simulink model "DiagramaFase2"  (R2024b)
settings: Solver=VariableStepAuto  StartTime=0.0  StopTime=5  RelTol=1e-3
settings Model: Creator=david  LastModifiedBy=david

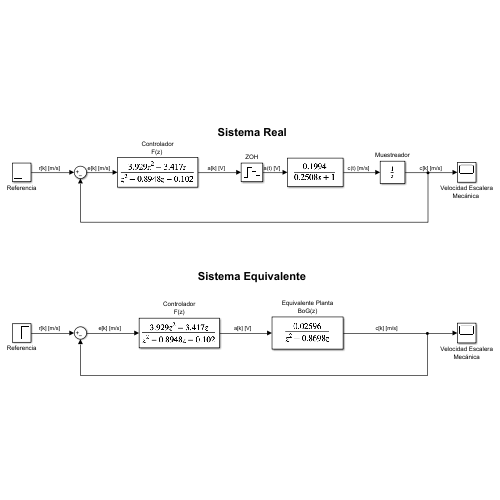
[thumbnail: Simulink's stored preview of the top-level diagram]
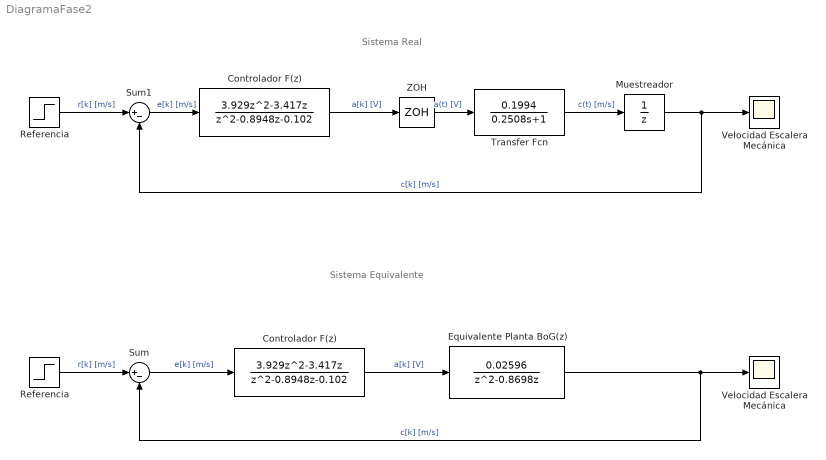
== system DiagramaFase2 ==
  note: Sistema Real
  note: Sistema Equivalente
  Controlador F(z) : DiscreteTransferFcn  Numerator=[3.929 -3.417 0]  Denominator=[1 -0.8948 -0.102]
  "Controlador F(z) " : DiscreteTransferFcn  Numerator=[3.929 -3.417 0]  Denominator=[1 -0.8948 -0.102]
  Equivalente Planta BoG(z) : DiscreteTransferFcn  Numerator=0.02596  Denominator=[1 -0.8698 0]
  Muestreador : DiscreteTransferFcn  Denominator=[1 0]
  Referencia : Step  Time=0  SampleTime=0.035
  "Referencia " : Step  Time=0  SampleTime=0.035
  Sum : Sum  Inputs=|+-
  Sum1 : Sum  Inputs=|+-
  Transfer Fcn : TransferFcn  Numerator=0.1994  Denominator=[0.2508 1]
  Velocidad Escalera Mecánica : Scope
  "Velocidad Escalera Mecánica " : Scope
  ZOH : ZeroOrderHold  SampleTime=0.035
  wires:
  Referencia/1 -> Sum/1  "r[k] [m/s]"
  Equivalente Planta BoG(z)/1 -> Sum/2, Velocidad Escalera Mecánica/1  "c[k] [m/s]"
  "Referencia "/1 -> Sum1/1  "r[k] [m/s]"
  "Controlador F(z) "/1 -> ZOH/1  "a[k] [V]"
  ZOH/1 -> Transfer Fcn/1  "a(t) [V]"
  Muestreador/1 -> "Velocidad Escalera Mecánica "/1, Sum1/2  "c[k] [m/s]"
  Sum1/1 -> "Controlador F(z) "/1  "e[k] [m/s]"
  Sum/1 -> Controlador F(z)/1  "e[k] [m/s]"
  Controlador F(z)/1 -> Equivalente Planta BoG(z)/1  "a[k] [V]"
  Transfer Fcn/1 -> Muestreador/1  "c(t) [m/s]"
